simulink model "Simulink_ISS_Model"  (R2019b)
settings: Solver=VariableStepAuto  StartTime=0.0  StopTime=60  RelTol=1e-3
values from neighbouring files (symbols this model uses):
  A = [     -den(2) 1;     -den(3) 0]    [Entire_System.m]
  B = [     num(2);     num(3)]    [Entire_System.m]
  C = [1 0]    [Entire_System.m]
  D = 0    [Entire_System.m]
  G = 1/(C*inv(eye(2)-A+B*K)*B)    [Entire_System.m]
  K = place(A,B,poles_desired)    [Entire_System.m]    (also in Motor_Code.m = [0.2641    0.6537])
  L = (place(A',C',poles))'    [Entire_System.m]
libraries: simulink x1
settings Model: Creator=Hamil  LastModifiedBy=Hamil
settings DataIOCC: ReturnWorkspaceOutputs=off
settings DebuggingCC: ArithmeticOperatorsInVariantConditions=warning
settings SFSimCC: SimUseLocalCustomCode=off  CustomCodeUndefinedFunction=UseInterfaceOnly
settings RTWCC: RTWUseLocalCustomCode=off

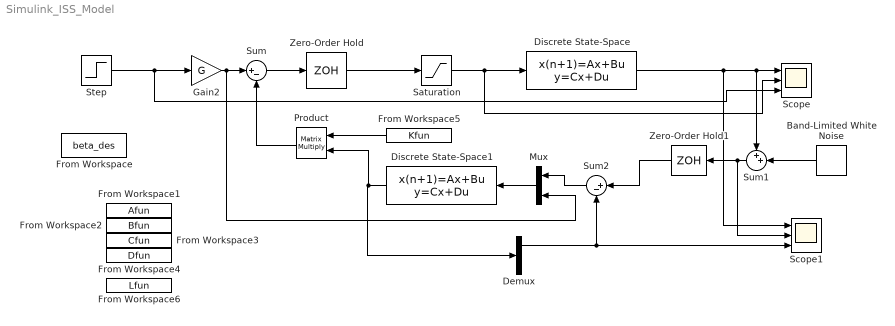
== system Simulink_ISS_Model ==
  Band-Limited White Noise : simulink/Sources/Band-Limited White Noise  Cov=[0.0000]  Ts=0.5  seed=[23341]
  Demux : Demux  Outputs=2
  Discrete State-Space : DiscreteStateSpace  A=A  B=B  C=C  D=D  SampleTime=0.5
  Discrete State-Space1 : DiscreteStateSpace  A=A-B*K  B=[L B]  C=[1 0;0 1]  D=[0 0;0 0]  SampleTime=-1
  From Workspace : FromWorkspace  VariableName=beta_des  OutDataTypeStr=double  SampleTime=.5
  From Workspace1 : FromWorkspace  VariableName=Afun  SampleTime=0.5  Interpolate=off  OutputAfterFinalValue=Holding final value
  From Workspace2 : FromWorkspace  VariableName=Bfun  SampleTime=0.5
  From Workspace3 : FromWorkspace  VariableName=Cfun  SampleTime=0.5
  From Workspace4 : FromWorkspace  VariableName=Dfun  SampleTime=0.5
  From Workspace5 : FromWorkspace  VariableName=Kfun  SampleTime=0.5
  From Workspace6 : FromWorkspace  VariableName=Lfun  SampleTime=0.5
  Gain2 : Gain  Gain=G
  Mux : Mux  Inputs=2
  Product : Product  Multiplication=Matrix(*)
  Saturation : Saturate  UpperLimit=1  LowerLimit=-1  OutMin=-1  OutMax=1
  Scope : Scope  NumInputPorts=3
  Scope1 : Scope  NumInputPorts=3
  Step : Step  SampleTime=0.5
  Sum : Sum  Inputs=|+-
  Sum1 : Sum  Inputs=++|
  Sum2 : Sum  Inputs=|+-
  Zero-Order Hold : ZeroOrderHold  SampleTime=0.5
  Zero-Order Hold1 : ZeroOrderHold  SampleTime=0.5
  wires:
  Sum/1 -> Zero-Order Hold/1
  Zero-Order Hold/1 -> Saturation/1
  Saturation/1 -> Scope/2, Discrete State-Space/1
  Discrete State-Space/1 -> Scope1/1, Sum1/1, Scope/1
  Gain2/1 -> Mux/2, Sum/1
  Step/1 -> Scope/3, Gain2/1
  Sum1/1 -> Scope1/2, Zero-Order Hold1/1
  Band-Limited White Noise/1 -> Sum1/2
  Zero-Order Hold1/1 -> Sum2/1
  Demux/1 -> Scope1/3, Sum2/2
  Product/1 -> Sum/2
  From Workspace5/1 -> Product/1
  Discrete State-Space1/1 -> Product/2, Demux/1
  Sum2/1 -> Mux/1
  Mux/1 -> Discrete State-Space1/1
